simulink model "DC_DC_SEPIC"  (R2023a)
settings: Solver=VariableStepAuto  StartTime=0.0  StopTime=10.0  RelTol=1e-3
libraries: spsSeriesRLCBranchLib x5, spsMeanLib x2, spsVoltageMeasurementLib x2, spsCurrentMeasurementLib x1, spsDCVoltageSourceLib x1, spsDiodeLib x1, spsGroundLib x1, spsMosfetLib x1, spspowerguiLib x1
settings Model: Creator=aakar  LastModifiedBy=aakar

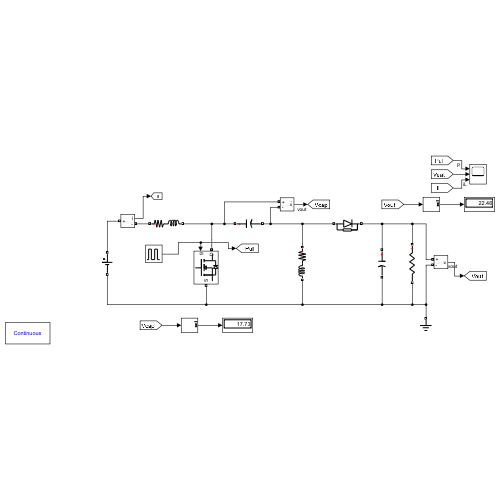
[thumbnail: Simulink's stored preview of the top-level diagram]
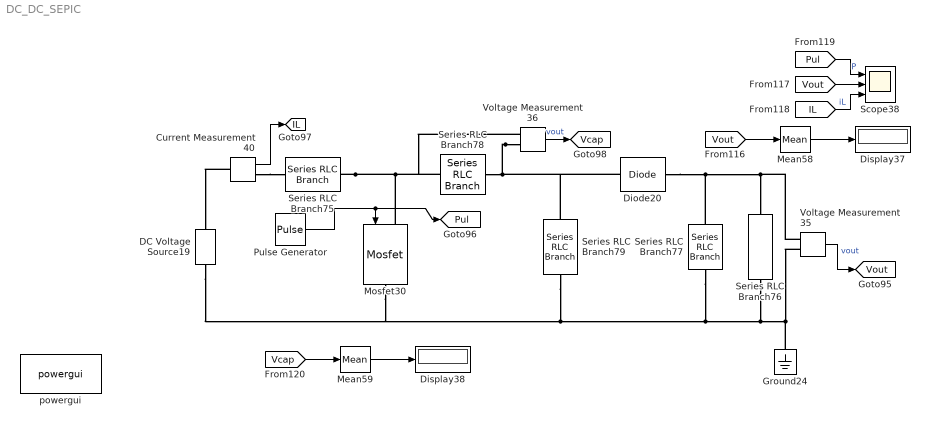
== system DC_DC_SEPIC ==
  Current Measurement40 : spsCurrentMeasurementLib/Current Measurement  PhasorSimulation=off  OutputType=Complex  PSBequivalent=0
  DC Voltage Source19 : spsDCVoltageSourceLib/DC Voltage Source  Amplitude=15  Measurements=None
  Diode20 : spsDiodeLib/Diode  Ron=1e-7  Lon=0  Vf=0  IC=0  UseSnubber=0  Rs=1e6  Cs=1e6  Measurements=off
  Display37 : Display
  Display38 : Display
  Ground24 : spsGroundLib/Ground  LConnTagsString=a
  Mean58 : spsMeanLib/Mean  Freq=10000  Vinit=0  Ts=0
  Mean59 : spsMeanLib/Mean  Freq=10000  Vinit=0  Ts=0
  Mosfet30 : spsMosfetLib/Mosfet  Ron=1e-7  Lon=0  Rd=1e-10  Vfd=0  IC=0  Rs=inf  Cs=0  Measurements=off
  Pulse Generator : DiscretePulseGenerator  PulseType=Time based  Period=200e-6  PulseWidth=60
  Scope38 : Scope  NumInputPorts=3
  Series RLC Branch75 : spsSeriesRLCBranchLib/Series RLC Branch  LConnTagsString=__new0  RConnTagsString=__new0  BranchType=RL  Resistance=0.000001  Inductance=1e-3  SetiL0=off  InitialCurrent=0  Capacitance=1e-6  Setx0=off  InitialVoltage=0  Measurements=None
  Series RLC Branch76 : spsSeriesRLCBranchLib/Series RLC Branch  LConnTagsString=__new0  RConnTagsString=__new0  BranchType=R  Resistance=22.5  Inductance=1e-3  SetiL0=off  InitialCurrent=0  Capacitance=1000e-6  Setx0=on  InitialVoltage=800  Measurements=None
  Series RLC Branch77 : spsSeriesRLCBranchLib/Series RLC Branch  LConnTagsString=__new0  RConnTagsString=__new0  BranchType=C  Resistance=0.001  Inductance=1e-3  SetiL0=off  InitialCurrent=0  Capacitance=220e-6  Setx0=off  InitialVoltage=800  Measurements=None
  Series RLC Branch78 : spsSeriesRLCBranchLib/Series RLC Branch  LConnTagsString=__new0  RConnTagsString=__new0  BranchType=C  Resistance=0.1  Inductance=1e-3  SetiL0=off  InitialCurrent=0  Capacitance=220e-6  Setx0=off  InitialVoltage=800  Measurements=None
  Series RLC Branch79 : spsSeriesRLCBranchLib/Series RLC Branch  LConnTagsString=__new0  RConnTagsString=__new0  BranchType=RL  Resistance=0.000001  Inductance=1e-3  SetiL0=off  InitialCurrent=0  Capacitance=1e-6  Setx0=off  InitialVoltage=0  Measurements=None
  Voltage Measurement35 : spsVoltageMeasurementLib/Voltage Measurement  PhasorSimulation=off  OutputType=Complex  PSBequivalent=0
  Voltage Measurement36 : spsVoltageMeasurementLib/Voltage Measurement  PhasorSimulation=off  OutputType=Complex  PSBequivalent=0
  powergui : spspowerguiLib/powergui  Priority=1  SimulationMode=Continuous  SampleTime=50e-6  frequency=60  Iterations=50  frequencyindice=0  Pbase=100e6  ErrMax=1e-4  UnitsV=kV  UnitsW=MW  buscounter=0  FunctionMessages=off  echomessages=off  EnableUseOfTLC=off  CurrentSourceSwitches=off  DisableSnubberDevices=off  DisableRonSwitches=off  DisableVfSwitches=off  DisplayEquations=off  AutomaticDiscreteSolvers=off  SolverType=Tustin/Backward Euler (TBE)  Interpol=off  ExternalGateDelay=off  methode=off  Ts=100  x0status=blocks  SPID=on  SwTol=0  HookPort=off  NonlinearTolerance=1e-4  nMaxIteration=100  ContinueOnMaxIteration=off  RestoreLinks=warning  ResistiveCurrentMeasurement=off  Frange=[0:2:500]  Ylog=off  Xlog=on  ShowGrid=off  save=off  variable=ZData  structure=0  ZoomFFT=off  StartTime=0.0  cycles=1  DisplayStyle=1  fundamental=60  FreqAxis=off  MaxFrequency=1000  frequencyindicesteady=1  RmsSteady=1  display=off
  tag scope: IL=global, Pul=global, Vcap=global, Vout=global
  wires:
  [Vout] -> Scope38/2
  [Vout] -> Mean58/1
  [Vcap] -> Mean59/1
  Voltage Measurement36/1 -> [Vcap]  "vout"
  [IL] -> Scope38/3  "iL"
  Mean59/1 -> Display38/1
  Mean58/1 -> Display37/1
  [Pul] -> Scope38/1  "P"
  Voltage Measurement35/1 -> [Vout]  "vout"
  Current Measurement40/1 -> [IL]
  Pulse Generator/1 -> Mosfet30/1, [Pul]
  connections:
  Voltage Measurement36/LConn2 -- Series RLC Branch78/RConn1 -- Diode20/LConn1 -- Series RLC Branch79/LConn1
  Series RLC Branch75/RConn1 -- Series RLC Branch78/LConn1 -- Voltage Measurement36/LConn1 -- Mosfet30/LConn1
  Series RLC Branch77/RConn1 -- Voltage Measurement35/LConn2 -- Ground24/LConn1 -- Series RLC Branch76/RConn1 -- DC Voltage Source19/LConn1 -- Mosfet30/RConn1 -- Series RLC Branch79/RConn1
  Diode20/RConn1 -- Voltage Measurement35/LConn1 -- Series RLC Branch76/LConn1 -- Series RLC Branch77/LConn1
  Current Measurement40/RConn1 -- Series RLC Branch75/LConn1
  Current Measurement40/LConn1 -- DC Voltage Source19/RConn1
